simulink model "Model_Equation"  (R2020a)
settings: Solver=FixedStepDiscrete  StartTime=0.0  StopTime=20  RelTol=1e-3
settings Model: Creator=DELL  LastModifiedBy=DELL
settings DataIOCC: SaveOutput=off  SaveTime=off

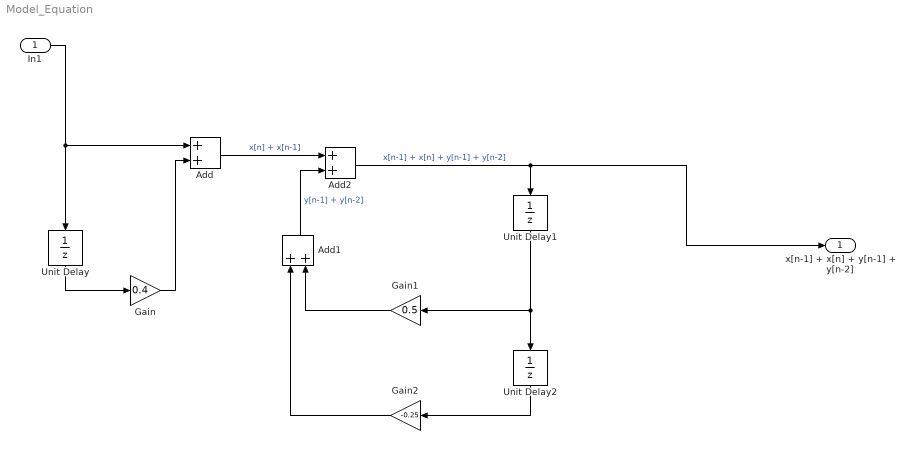
== system Model_Equation ==
  In1 : Inport  OutDataTypeStr=double  PortDimensions=1  SampleTime=0
  Add : Sum
  Add1 : Sum
  Add2 : Sum
  Gain : Gain  Gain=0.4
  Gain1 : Gain  Gain=0.5
  Gain2 : Gain  Gain=-0.25
  Unit Delay : UnitDelay  SampleTime=-1  HasFrameUpgradeWarning=on
  Unit Delay1 : UnitDelay  SampleTime=-1  HasFrameUpgradeWarning=on
  Unit Delay2 : UnitDelay  SampleTime=-1  HasFrameUpgradeWarning=on
  x[n-1] + x[n] + y[n-1] + y[n-2] : Outport  OutDataTypeStr=double  PortDimensions=1  SampleTime=0
  wires:
  Unit Delay/1 -> Gain/1
  Add2/1 -> Unit Delay1/1, x[n-1] + x[n] + y[n-1] + y[n-2]/1  "x[n-1] + x[n] + y[n-1] + y[n-2]"
  Gain2/1 -> Add1/1
  Add1/1 -> Add2/2  "y[n-1] + y[n-2]"
  In1/1 -> Add/1, Unit Delay/1
  Unit Delay1/1 -> Unit Delay2/1, Gain1/1
  Unit Delay2/1 -> Gain2/1
  Gain1/1 -> Add1/2
  Add/1 -> Add2/1  "x[n] + x[n-1]"
  Gain/1 -> Add/2
